simulink model "lqr_swarm"  (R2025a)
settings: Solver=VariableStepAuto  StartTime=0.0  StopTime=250  RelTol=1e-3
values from neighbouring files (symbols this model uses):
  A = [0 0 0 0 0 0 -g 0 0 0 0 0 ... (first row only)    [analysis.m]    (also in constants.m; hinf_design.m; linear_nonlinear_comparison.m)
  A1 = A    [analysis.m]
  A2 = A    [analysis.m]
  A3 = A    [analysis.m]
  B = [0 0 0 0 ... (first row only)    [analysis.m]    (also in constants.m; hinf_design.m; linear_nonlinear_comparison.m)
  B1 = B    [analysis.m]
  B2 = B    [analysis.m]
  B3 = B    [analysis.m]
  simcase = STABILIZE    (= 4)    [analysis.m]    (also in sweep_ballistic_envelope.m; sweep_landing_centroid.m)
  x0_step = [2; 4; 10]    [analysis.m]    (also in sweep_ballistic_envelope.m; sweep_landing_centroid.m)
  xf = [0; 0; 0]    [analysis.m]    (also in sweep_ballistic_envelope.m; sweep_landing_centroid.m)
  xi = [vel0; rotvel0; rot0; x0]    [analysis.m]    (also in ballistic_deploy_state.m = [vel0; rotvel0; theta0; phi0; psi0; pos_nwu]; dsmc_constraints.m = (1 - k_xi) .* xi + delta_u; forensic_envelope.m = ballistic_deploy_state(dp(1:3), dp(4:6), dp(7:9), dp(10:12)); sweep_ballistic_envelope.m = ballistic_deploy_state(deploy_point(1:3), deploy_point(4:6),)
libraries: uavutilslib x1
settings Model: SimulationMode=rapid-accelerator  ExtModeTrigDuration=100  Creator=johnpye  LastModifiedBy=johnpye

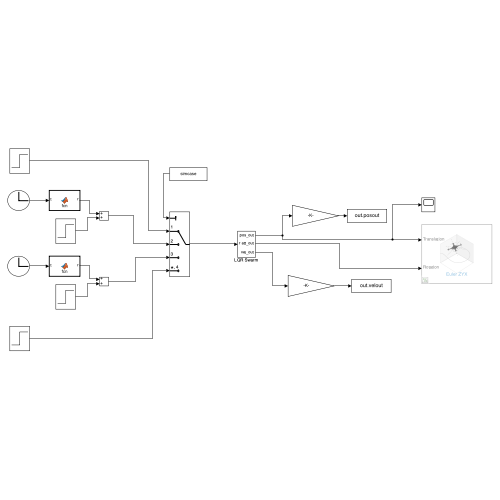
[thumbnail: Simulink's stored preview of the top-level diagram]
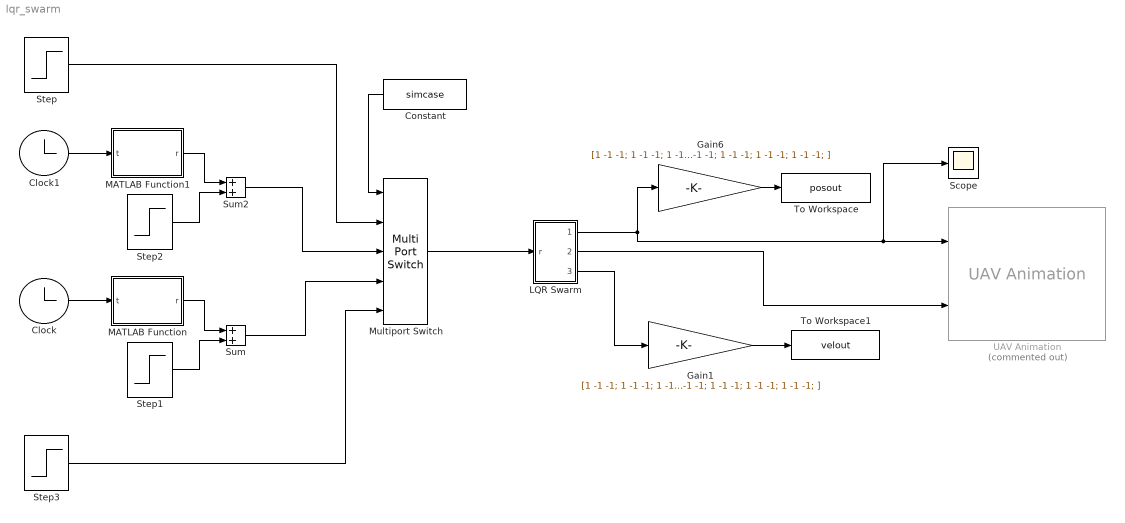
== system lqr_swarm ==
  Clock : Clock
  Clock1 : Clock
  Constant : Constant  Value=simcase
  Gain1 : Gain  Gain=[1 -1 -1; 1 -1 -1; 1 -1 -1; 1 -1 -1; 1 -1 -1; 1 -1 -1; 1 -1 -1; 1 -1 -1; 1 -1 -1; 1 -1 -1; ]
  Gain6 : Gain  Gain=[1 -1 -1; 1 -1 -1; 1 -1 -1; 1 -1 -1; 1 -1 -1; 1 -1 -1; 1 -1 -1; 1 -1 -1; 1 -1 -1; 1 -1 -1; ]
  LQR Swarm : Subsystem
  MATLAB Function : MATLAB Function  TreatAsAtomicUnit=on
  MATLAB Function1 : MATLAB Function  TreatAsAtomicUnit=on
  Multiport Switch : MultiPortSwitch  Inputs=4  SaturateOnIntegerOverflow=off  InputSameDT=off
  Scope : Scope
      settings: ActiveDisplayYMinimum=-13.381543333511724  ActiveDisplayYMaximum=9.2646159259457477
  Step : Step  Time=0  Before=x0_step  After=xf  SampleTime=0  VectorParams1D=off
  Step1 : Step  Time=0  Before=[0; 0; 0]  After=[0; 0; 10]  SampleTime=0  VectorParams1D=off
  Step2 : Step  Time=0  Before=[0; 0; 0]  After=[0; 0; 10]  SampleTime=0  VectorParams1D=off
  Step3 : Step  Time=0  Before=xi(10:12,:)  After=[xi(10:11,:);0]  SampleTime=0  VectorParams1D=off
  Sum : Sum
  Sum2 : Sum
  To Workspace : ToWorkspace  VariableName=posout  SaveFormat=Timeseries  SampleTime=-1
  To Workspace1 : ToWorkspace  VariableName=velout  SaveFormat=Timeseries  SampleTime=-1
  UAV Animation : uavutilslib/UAV Animation  Commented=on  NumUAV=10  DynamicUAVConfig=off  UAVType=Multirotor  UAVSize=1  UAVColor=[1 0 0]  UAVTrajectoryAlpha=1  InertialZDirection=Down  RotationFormat=Euler ZYX  DrawMarkers=off  SampleTime=-1
  wires:
  LQR Swarm/2(att_out) -> UAV Animation/2
  LQR Swarm/1(pos_out) -> Scope/1, UAV Animation/1, Gain6/1
  Multiport Switch/1 -> LQR Swarm/1(r)
  Gain6/1 -> To Workspace/1
  Gain1/1 -> To Workspace1/1
  LQR Swarm/3(vel_out) -> Gain1/1
  Step3/1 -> Multiport Switch/5
  Clock1/1 -> MATLAB Function1/1(t)
  MATLAB Function/1(r) -> Sum/1
  Constant/1 -> Multiport Switch/1
  Sum/1 -> Multiport Switch/4
  Step/1 -> Multiport Switch/2
  Step1/1 -> Sum/2
  Clock/1 -> MATLAB Function/1(t)
  Sum2/1 -> Multiport Switch/3
  Step2/1 -> Sum2/2
  MATLAB Function1/1(r) -> Sum2/1

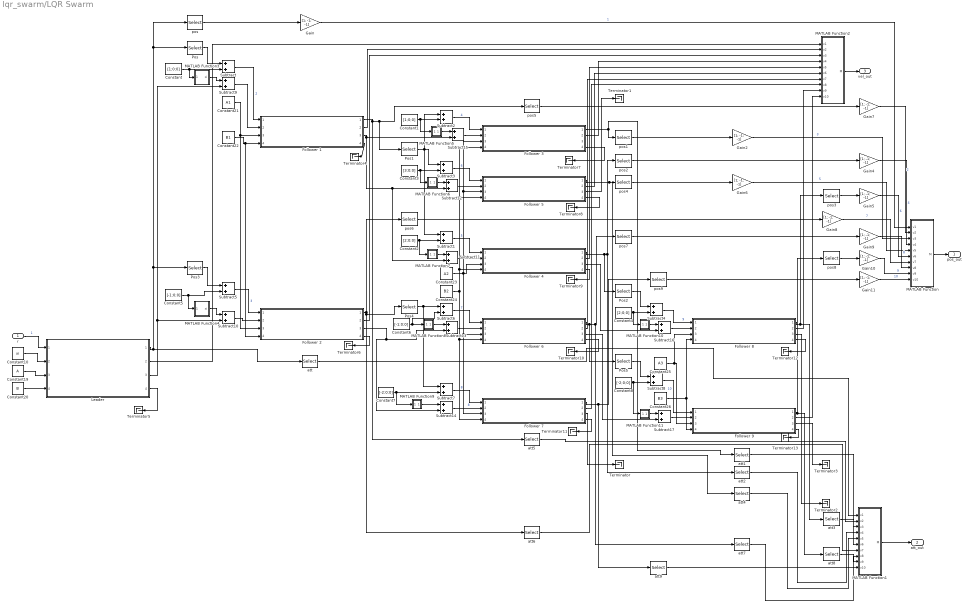
== system lqr_swarm/LQR Swarm ==
  r : Inport
  Constant : Constant  Value=[1;0;0]
  Constant1 : Constant  Value=[1;0;0]
  Constant10 : Constant  Value=xi
  Constant19 : Constant  Value=A
  Constant2 : Constant  Value=[2;0;0]
  Constant20 : Constant  Value=B
  Constant21 : Constant  Value=A1
  Constant22 : Constant  Value=B1
  Constant23 : Constant  Value=A2
  Constant24 : Constant  Value=B2
  Constant25 : Constant  Value=A3
  Constant26 : Constant  Value=B3
  Constant3 : Constant  Value=[3;0;0]
  Constant4 : Constant  Value=[2;0;0]
  Constant5 : Constant  Value=[-1;0;0]
  Constant6 : Constant  Value=[-1;0;0]
  Constant7 : Constant  Value=[-2;0;0]
  Constant8 : Constant  Value=[-2;0;0]
  Follower {1..9} (9 alike) : Subsystem  ReferencedSubsystem=discrete_lqr_controller
  Gain{,2,4..11} (10 alike) : Gain  Gain=[1; -1; -1]
  Leader : Subsystem  ReferencedSubsystem=discrete_lqr_controller
  MATLAB Function : MATLAB Function  TreatAsAtomicUnit=on
  MATLAB Function1 : MATLAB Function  TreatAsAtomicUnit=on
  MATLAB Function10 : MATLAB Function  TreatAsAtomicUnit=on
  MATLAB Function11 : MATLAB Function  TreatAsAtomicUnit=on
  MATLAB Function2 : MATLAB Function  TreatAsAtomicUnit=on
  MATLAB Function3 : MATLAB Function  TreatAsAtomicUnit=on
  MATLAB Function4 : MATLAB Function  TreatAsAtomicUnit=on
  MATLAB Function5 : MATLAB Function  TreatAsAtomicUnit=on
  MATLAB Function6 : MATLAB Function  TreatAsAtomicUnit=on
  MATLAB Function7 : MATLAB Function  TreatAsAtomicUnit=on
  MATLAB Function8 : MATLAB Function  TreatAsAtomicUnit=on
  MATLAB Function9 : MATLAB Function  TreatAsAtomicUnit=on
  Pos{,1..5} (6 alike) : Selector  InputPortWidth=12  IndexOptions=Index vector (dialog)  Indices=[10 11 12]  OutputSizes=1
  Subtract{,1..17} (18 alike) : Sum
  Terminator{,1..13} (14 alike) : Terminator
  att{,1..9} (10 alike) : Selector  InputPortWidth=12  IndexOptions=Index vector (dialog)  Indices=[7 8 9]  OutputSizes=1
  pos{,1..9} (10 alike) : Selector  InputPortWidth=12  IndexOptions=Index vector (dialog)  Indices=[10 11 12]  OutputSizes=1
  pos_out : Outport
  att_out : Outport  Port=2
  vel_out : Outport  Port=3
  wires:
  MATLAB Function1/1(M) -> att_out/1
  Gain11/1 -> MATLAB Function/10(v10)  "10"
  Gain10/1 -> MATLAB Function/9(v9)  "9"
  Gain9/1 -> MATLAB Function/8(v8)  "8"
  Gain5/1 -> MATLAB Function/6(v6)  "6"
  Gain4/1 -> MATLAB Function/4(v4)  "4"
  Gain7/1 -> MATLAB Function/2(v2)  "2"
  att4/1 -> MATLAB Function1/5(v5)
  att8/1 -> MATLAB Function1/9(v9)
  Pos3/1 -> Subtract5/1
  att3/1 -> MATLAB Function1/6(v6)
  Leader/1 -> Pos/1, pos/1, Pos3/1, att/1
  Follower 3/1 -> pos1/1, att1/1
  Gain8/1 -> MATLAB Function/7(v7)  "7"
  Pos1/1 -> Subtract2/1, Subtract1/1, Subtract3/1
  pos3/1 -> Gain5/1
  MATLAB Function/1(M) -> pos_out/1
  MATLAB Function2/1(M) -> vel_out/1
  Constant26/1 -> Follower 8/4, Follower 9/4
  att7/1 -> MATLAB Function1/8(v8)
  Follower 9/1 -> pos8/1, att8/1
  Follower 8/2 -> MATLAB Function2/9(v9)
  Follower 8/1 -> pos3/1, att3/1
  pos1/1 -> Gain2/1
  Subtract16/1 -> Follower 8/2
  Follower 2/3 -> Subtract13/2, Subtract14/2
  att1/1 -> MATLAB Function1/3(v3)
  Subtract4/1 -> Follower 8/1  "9"
  Constant4/1 -> Subtract4/2, MATLAB Function10/1(offset)
  att9/1 -> MATLAB Function1/10(v10)
  att5/1 -> MATLAB Function1/2(v2)
  pos7/1 -> Gain9/1
  Gain/1 -> MATLAB Function/1(v1)  "1"
  pos2/1 -> Gain4/1
  pos8/1 -> Gain10/1
  att6/1 -> MATLAB Function1/7(v7)
  Constant8/1 -> Subtract8/2, MATLAB Function11/1(offset)
  Constant19/1 -> Leader/3
  Pos2/1 -> Subtract4/1
  Constant2/1 -> Subtract1/2, MATLAB Function7/1(offset)
  Subtract17/1 -> Follower 9/2
  Follower 6/2 -> MATLAB Function2/7(v7)
  Follower 8/3 -> Terminator2/1
  Follower 6/1 -> pos7/1, att7/1, Pos5/1
  Follower 4/2 -> MATLAB Function2/5(v5)
  Subtract13/1 -> Follower 6/2
  Follower 2/2 -> MATLAB Function2/3(v3)
  Subtract15/1 -> Follower 3/2
  Constant25/1 -> Follower 8/3, Follower 9/3
  Follower 4/3 -> Subtract16/2
  Constant24/1 -> Follower 6/4, Follower 7/4, Follower 5/4, Follower 3/4, Follower 4/4
  Follower 5/3 -> Terminator1/1
  att/1 -> MATLAB Function1/1(v1)
  Follower 7/2 -> MATLAB Function2/8(v8)
  Follower 5/1 -> pos4/1, att4/1
  Subtract14/1 -> Follower 7/2  "8"
  Constant7/1 -> Subtract7/2, MATLAB Function9/1(offset)
  Subtract7/1 -> Follower 7/1  "8"
  Follower 9/3 -> Terminator3/1
  Subtract6/1 -> Follower 6/1  "7"
  Follower 6/3 -> Subtract17/2
  Subtract1/1 -> Follower 4/1  "5"
  Subtract3/1 -> Follower 5/1  "6"
  Subtract2/1 -> Follower 3/1  "4"
  Follower 2/1 -> Pos4/1, att6/1, pos6/1
  Follower 7/3 -> Terminator/1
  Follower 4/1 -> pos2/1, att2/1, Pos2/1
  Follower 5/2 -> MATLAB Function2/6(v6)
  Pos4/1 -> Subtract7/1, Subtract6/1
  pos6/1 -> Gain8/1
  Leader/2 -> MATLAB Function2/1(v1)
  Follower 3/2 -> MATLAB Function2/4(v4)
  Subtract11/1 -> Follower 4/2
  Constant3/1 -> Subtract3/2, MATLAB Function6/1(offset)
  pos5/1 -> Gain7/1
  Subtract10/1 -> Follower 2/2
  Constant23/1 -> Follower 6/3, Follower 7/3, Follower 5/3, Follower 3/3, Follower 4/3
  Follower 1/3 -> Subtract11/2, Subtract12/2, Subtract15/2
  Subtract12/1 -> Follower 5/2
  Constant/1 -> MATLAB Function3/1(offset), Subtract/2
  Follower 1/2 -> MATLAB Function2/2(v2)
  Constant21/1 -> Follower 1/3, Follower 2/3
  Constant1/1 -> Subtract2/2, MATLAB Function5/1(offset)
  Pos5/1 -> Subtract8/1
  Subtract5/1 -> Follower 2/1  "3"
  Subtract9/1 -> Follower 1/2
  Constant22/1 -> Follower 1/4, Follower 2/4
  Subtract/1 -> Follower 1/1  "2"
  Follower 7/1 -> att9/1, pos9/1
  Constant6/1 -> MATLAB Function8/1(offset), Subtract6/2
  Constant5/1 -> Subtract5/2, MATLAB Function4/1(offset)
  Follower 9/2 -> MATLAB Function2/10(v10)
  Pos/1 -> Subtract/1
  pos4/1 -> Gain6/1
  Follower 1/1 -> att5/1, Pos1/1, pos5/1
  r/1 -> Leader/1  "1"
  Gain6/1 -> MATLAB Function/5(v5)  "5"
  pos/1 -> Gain/1
  att2/1 -> MATLAB Function1/4(v4)
  Gain2/1 -> MATLAB Function/3(v3)  "3"
  Subtract8/1 -> Follower 9/1  "10"
  pos9/1 -> Gain11/1
  Constant20/1 -> Leader/4
  Leader/3 -> Subtract10/2, Subtract9/2
  Constant10/1 -> Leader/2
  MATLAB Function3/1(xi) -> Subtract9/1
  MATLAB Function4/1(xi) -> Subtract10/1
  MATLAB Function5/1(xi) -> Subtract15/1
  MATLAB Function6/1(xi) -> Subtract12/1
  MATLAB Function7/1(xi) -> Subtract11/1
  MATLAB Function8/1(xi) -> Subtract13/1
  MATLAB Function9/1(xi) -> Subtract14/1
  MATLAB Function10/1(xi) -> Subtract16/1
  MATLAB Function11/1(xi) -> Subtract17/1
  Leader/4 -> Terminator5/1
  Follower 1/4 -> Terminator4/1
  Follower 2/4 -> Terminator6/1
  Follower 3/4 -> Terminator7/1
  Follower 5/4 -> Terminator8/1
  Follower 4/4 -> Terminator9/1
  Follower 6/4 -> Terminator10/1
  Follower 7/4 -> Terminator11/1
  Follower 8/4 -> Terminator12/1
  Follower 9/4 -> Terminator13/1

== matlab function lqr_swarm/LQR Swarm/MATLAB Function7 ==
  data: offset input; xi output
function xi = init(offset)

xi = [zeros(9,1); offset];

== matlab function lqr_swarm/LQR Swarm/MATLAB Function8 ==
  data: offset input; xi output
function xi = init(offset)

xi = [zeros(9,1); offset];

== matlab function lqr_swarm/LQR Swarm/MATLAB Function9 ==
  data: offset input; xi output
function xi = init(offset)

xi = [zeros(9,1); offset];

== matlab function lqr_swarm/LQR Swarm/MATLAB Function10 ==
  data: offset input; xi output
function xi = init(offset)

xi = [zeros(9,1); offset];

== matlab function lqr_swarm/LQR Swarm/MATLAB Function11 ==
  data: offset input; xi output
function xi = init(offset)

xi = [zeros(9,1); offset];

== matlab function lqr_swarm/LQR Swarm/MATLAB Function2 ==
  data: v1 input; M output; v2 input; v3 input; v4 input; v5 input; v6 input; v7 input; v8 input; v9 input; v10 input
function M = fcn(v1, v2, v3, v4, v5, v6, v7, v8, v9, v10)

v1 = reshape(v1, [1, 3]);
v2 = reshape(v2, [1, 3]);
v3 = reshape(v3, [1, 3]);
v4 = reshape(v4, [1, 3]);
v5 = reshape(v5, [1, 3]);
v6 = reshape(v6, [1, 3]);
v7 = reshape(v7, [1, 3]);
v8 = reshape(v8, [1, 3]);
v9 = reshape(v9, [1, 3]);
v10 = reshape(v10, [1, 3]);

M = [v1; v2; v3; v4; v5; v6; v7; v8; v9; v10];

== matlab function lqr_swarm/LQR Swarm/MATLAB Function3 ==
  data: offset input; xi output
function xi = init(offset)

xi = [zeros(9,1); offset];

== matlab function lqr_swarm/LQR Swarm/MATLAB Function4 ==
  data: offset input; xi output
function xi = init(offset)

xi = [zeros(9,1); offset];

== matlab function lqr_swarm/MATLAB Function ==
  data: t input; r output
function r = fcn(t)

r = [0.05*t*cos(2*pi*0.05*t); 0.05*t*sin(2*pi*0.05*t); 0];

== matlab function lqr_swarm/MATLAB Function1 ==
  data: t input; r output
function r = fcn(t)

r = [-0.25*cos(2*pi*0.05*t); 10*sin(2*pi*0.05*t)*cos(2*pi*0.05*t); 0];

== matlab function lqr_swarm/LQR Swarm/MATLAB Function ==
  data: v1 input; M output; v2 input; v3 input; v4 input; v5 input; v6 input; v7 input; v8 input; v9 input; v10 input
function M = fcn(v1, v2, v3, v4, v5, v6, v7, v8, v9, v10)

v1 = reshape(v1, [1, 3]);
v2 = reshape(v2, [1, 3]);
v3 = reshape(v3, [1, 3]);
v4 = reshape(v4, [1, 3]);
v5 = reshape(v5, [1, 3]);
v6 = reshape(v6, [1, 3]);
v7 = reshape(v7, [1, 3]);
v8 = reshape(v8, [1, 3]);
v9 = reshape(v9, [1, 3]);
v10 = reshape(v10, [1, 3]);

M = [v1; v2; v3; v4; v5; v6; v7; v8; v9; v10];

== matlab function lqr_swarm/LQR Swarm/MATLAB Function1 ==
  data: v1 input; M output; v2 input; v3 input; v4 input; v5 input; v6 input; v7 input; v8 input; v9 input; v10 input
function M = fcn(v1, v2, v3, v4, v5, v6, v7, v8, v9, v10)

v1 = reshape(v1, [1, 3]);
v2 = reshape(v2, [1, 3]);
v3 = reshape(v3, [1, 3]);
v4 = reshape(v4, [1, 3]);
v5 = reshape(v5, [1, 3]);
v6 = reshape(v6, [1, 3]);
v7 = reshape(v7, [1, 3]);
v8 = reshape(v8, [1, 3]);
v9 = reshape(v9, [1, 3]);
v10 = reshape(v10, [1, 3]);

M = [v1; v2; v3; v4; v5; v6; v7; v8; v9; v10];

== matlab function lqr_swarm/LQR Swarm/MATLAB Function5 ==
  data: offset input; xi output
function xi = init(offset)

xi = [zeros(9,1); offset];

== matlab function lqr_swarm/LQR Swarm/MATLAB Function6 ==
  data: offset input; xi output
function xi = init(offset)

xi = [zeros(9,1); offset];
